simulink model "InversorDiesel"  (R2017a)
settings: Solver=VariableStepAuto  StartTime=0.0  StopTime=10.0  MaxStep=1e-4  RelTol=1e-3
values from neighbouring files (symbols this model uses):
  C1 = 1.1e-6    (= 1.1e-06)    [sistemacontrolado.m]
  L1 = 4.5e-3    (= 0.0045)    [sistemacontrolado.m]
  La = 3e-3    (= 0.003)    [sistemacontrolado.m]
  R1 = 1    [sistemacontrolado.m]
libraries: powerlib x17, instrumentlib x3, powerlib_extras x1, simulink x1
settings Model: Creator=MarioAndres  LastModifiedBy=Diego

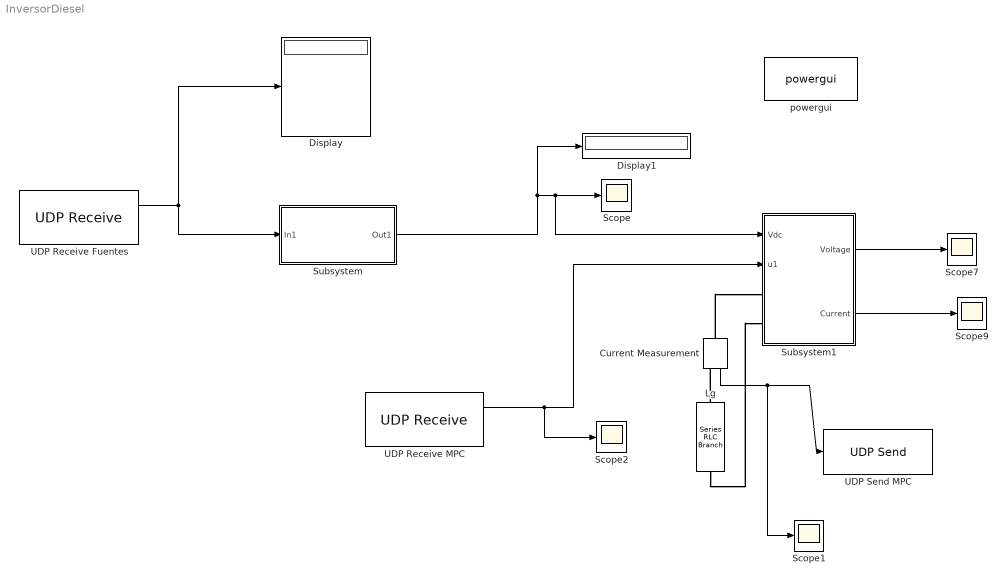
== system InversorDiesel ==
  Current Measurement : powerlib/Measurements/Current Measurement  PhasorSimulation=off  OutputType=Complex  PSBequivalent=0
  Display : Display
  Display1 : Display
  Lg : powerlib/Elements/Series RLC Branch  LConnTagsString=__new0  RConnTagsString=__new0  BranchType=L  Resistance=R1  Inductance=0.003  SetiL0=off  InitialCurrent=0  Capacitance=1e-6  Setx0=off  InitialVoltage=0  Measurements=None
  Scope{,1..2,7,9} (5 alike) : Scope
  Subsystem : Subsystem
  Subsystem1 : Subsystem
  UDP Receive Fuentes : instrumentlib/UDP Receive  Host=169.254.205.197  Port=51007  LocalPort=51006  DataSize="[6  1]"  EnableBlockingMode=off  Timeout=1  SampleTime=1  DataType=uint8  ByteOrder=BigEndian
      settings: SourceProductName=Instrument Control Toolbox
  UDP Receive MPC : instrumentlib/UDP Receive  Host=169.254.26.15  Port=51005  LocalPort=51004  DataSize="[6  1]"  EnableBlockingMode=off  Timeout=1  SampleTime=1  DataType=uint8  ByteOrder=BigEndian
      settings: SourceProductName=Instrument Control Toolbox
  UDP Send MPC : instrumentlib/UDP Send  Priority=2  Host=169.254.26.15  Port=51005  LocalPort=51004  EnableBlockingMode=on  ByteOrder=BigEndian
      settings: SourceProductName=Instrument Control Toolbox
  powergui : powerlib/powergui  SimulationMode=Continuous  SampleTime=1/60/10000  frequency=60  Iterations=50  frequencyindice=0  Pbase=100e6  ErrMax=1e-4  UnitsV=kV  UnitsW=MW  buscounter=0  FunctionMessages=off  echomessages=off  EnableUseOfTLC=off  CurrentSourceSwitches=off  DisableSnubberDevices=off  DisableRonSwitches=off  DisableVfSwitches=off  DisplayEquations=off  SolverType=Tustin/Backward Euler (TBE)  Interpol=off  ExternalGateDelay=off  methode=off  Ts=100  x0status=blocks  SPID=on  SwTol=0  HookPort=off  RestoreLinks=warning  ResistiveCurrentMeasurement=off  Frange=[0:2:500]  Ylog=off  Xlog=on  ShowGrid=off  save=off  variable=ZData  structure=sps1phPWM1_str  ZoomFFT=on  StartTime=0.1-2/60  cycles=2  DisplayStyle=1  fundamental=60  FreqAxis=off  MaxFrequency=5000  frequencyindicesteady=1  RmsSteady=1  display=off
  wires:
  UDP Receive Fuentes/1 -> Subsystem/1(In1), Display/1
  Subsystem1/1(Voltage) -> Scope7/1
  Subsystem1/2(Current) -> Scope9/1
  UDP Receive MPC/1 -> Scope2/1, Subsystem1/2(u1)
  Current Measurement/1 -> Scope1/1, UDP Send MPC/1
  Subsystem/1(Out1) -> Display1/1, Subsystem1/1(Vdc), Scope/1
  connections:
  Current Measurement/LConn1 -- Subsystem1/LConn1
  Lg/RConn1 -- Current Measurement/RConn1
  Lg/LConn1 -- Subsystem1/LConn2

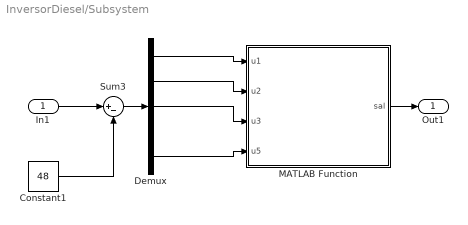
== system InversorDiesel/Subsystem ==
  In1 : Inport
  Constant1 : Constant  Value=48
  Demux : Demux  Outputs=5
  MATLAB Function : MATLAB Function  TreatAsAtomicUnit=on
  Sum3 : Sum  Inputs=|+-
  Out1 : Outport
  wires:
  Sum3/1 -> Demux/1
  In1/1 -> Sum3/1
  Constant1/1 -> Sum3/2
  Demux/1 -> MATLAB Function/1(u1)
  Demux/2 -> MATLAB Function/2(u2)
  Demux/3 -> MATLAB Function/3(u3)
  Demux/5 -> MATLAB Function/4(u5)
  MATLAB Function/1(sal) -> Out1/1

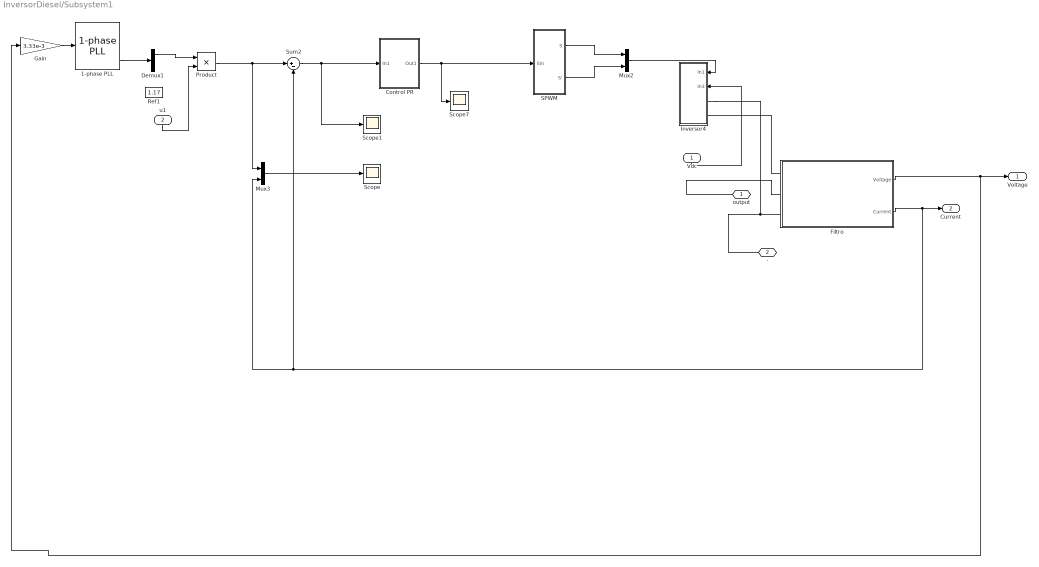
== system InversorDiesel/Subsystem1 ==
  Vdc : Inport
  u1 : Inport  Port=2
  1-phase PLL : powerlib_extras/Control  Blocks/1-phase PLL  Par_Init=[0 60]  ParK=[ 180 3200 1 ]  AGC=off
  Control PR : Subsystem
  Demux1 : Demux  Outputs=2
  Filtro : Subsystem
  Gain : Gain  Gain=3.33e-3
  Inversor4 : Subsystem
  Mux2 : Mux  Inputs=2
  Mux3 : Mux  Inputs=2
  Product : Product
  Ref1 : Constant  Value=1.17
  SPWM : Subsystem
  Scope : Scope
  Scope1 : Scope
  Scope7 : Scope
  Sum2 : Sum  Inputs=|+-
  output : PMIOPort  Port=1  Side=Left
  - : PMIOPort  Port=2  Side=Left
  Voltage : Outport
  Current : Outport  Port=2
  wires:
  Filtro/2(Current) -> Mux3/2, Sum2/2, Current/1
  Filtro/1(Voltage) -> Gain/1, Voltage/1
  1-phase PLL/3 -> Demux1/1
  Gain/1 -> 1-phase PLL/1
  Mux3/1 -> Scope/1
  Product/1 -> Mux3/1, Sum2/1
  Demux1/1 -> Product/1
  SPWM/1(S) -> Mux2/1
  SPWM/2(S') -> Mux2/2
  Mux2/1 -> Inversor4/1(In1)
  Vdc/1 -> Inversor4/2(In3)
  Control PR/1(Out1) -> Scope7/1, SPWM/1(Sin)
  Sum2/1 -> Scope1/1, Control PR/1(In1)
  u1/1 -> Product/2
  connections:
  output/RConn1 -- Filtro/LConn2
  -/RConn1 -- Inversor4/LConn1 -- Filtro/LConn3
  Filtro/LConn1 -- Inversor4/LConn2

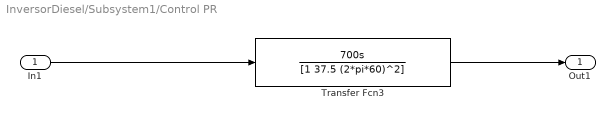
== system InversorDiesel/Subsystem1/Control PR ==
  In1 : Inport
  Transfer Fcn3 : TransferFcn  Numerator=[700 0]  Denominator=[1 37.5 (2*pi*60)^2]
  Out1 : Outport
  wires:
  In1/1 -> Transfer Fcn3/1
  Transfer Fcn3/1 -> Out1/1

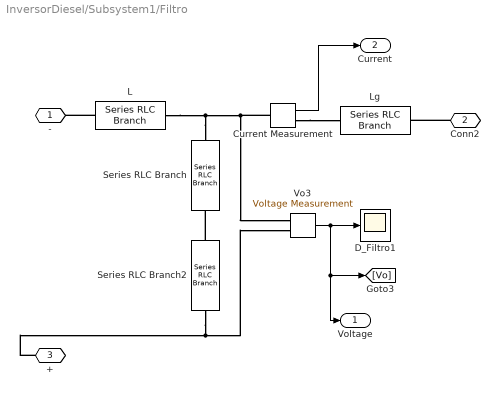
== system InversorDiesel/Subsystem1/Filtro ==
  Current Measurement : powerlib/Measurements/Current Measurement  PhasorSimulation=off  OutputType=Complex  PSBequivalent=0
  D_Filtro1 : Scope
  L : powerlib/Elements/Series RLC Branch  LConnTagsString=__new0  RConnTagsString=__new0  BranchType=RL  Resistance=0.01  Inductance=La  SetiL0=off  InitialCurrent=0  Capacitance=1e-6  Setx0=off  InitialVoltage=0  Measurements=None
  Lg : powerlib/Elements/Series RLC Branch  LConnTagsString=__new0  RConnTagsString=__new0  BranchType=RL  Resistance=R1  Inductance=L1  SetiL0=off  InitialCurrent=0  Capacitance=1e-6  Setx0=off  InitialVoltage=0  Measurements=None
  Series RLC Branch : powerlib/Elements/Series RLC Branch  LConnTagsString=__new0  RConnTagsString=__new0  BranchType=C  Resistance=10  Inductance=25e-3  SetiL0=off  InitialCurrent=0  Capacitance=C1  Setx0=on  InitialVoltage=0  Measurements=None
  Series RLC Branch2 : powerlib/Elements/Series RLC Branch  LConnTagsString=__new0  RConnTagsString=__new0  BranchType=R  Resistance=0.1  Inductance=25e-3  SetiL0=off  InitialCurrent=0  Capacitance=5.30e-3  Setx0=off  InitialVoltage=0  Measurements=None
  Vo3 : powerlib/Measurements/Voltage Measurement  PhasorSimulation=off  OutputType=Complex  PSBequivalent=0
  - : PMIOPort  Port=1  Side=Left
  Conn2 : PMIOPort  Port=2  Side=Left
  + : PMIOPort  Port=3  Side=Left
  Voltage : Outport
  Current : Outport  Port=2
  wires:
  Vo3/1 -> D_Filtro1/1, Voltage/1, [Vo]
  Current Measurement/1 -> Current/1
  connections:
  L/LConn1 -- -/RConn1
  Series RLC Branch/LConn1 -- Current Measurement/LConn1 -- Vo3/LConn1 -- L/RConn1
  Series RLC Branch2/LConn1 -- Series RLC Branch/RConn1
  Current Measurement/RConn1 -- Lg/LConn1
  Series RLC Branch2/RConn1 -- +/RConn1 -- Vo3/LConn2
  Conn2/RConn1 -- Lg/RConn1

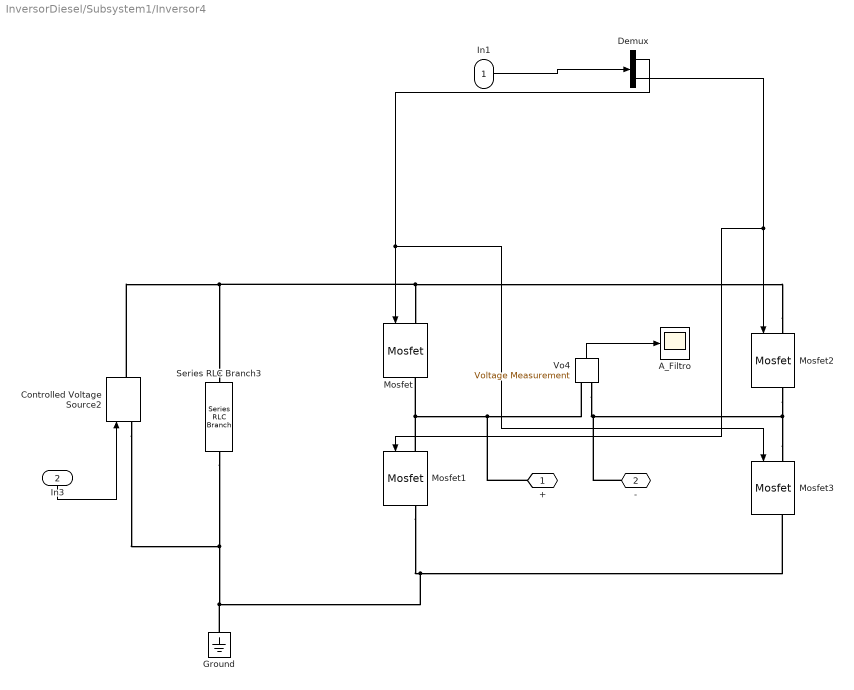
== system InversorDiesel/Subsystem1/Inversor4 ==
  In1 : Inport
  In3 : Inport  Port=2
  A_Filtro : Scope
  Controlled Voltage Source2 : powerlib/Electrical Sources/Controlled Voltage Source  Initialize=on  Source_Type=DC  Amplitude=0  Phase=0  Frequency=0  Measurements=None
  Demux : Demux  Outputs=2
  Ground : powerlib/Elements/Ground  LConnTagsString=a
  Mosfet{,1..3} (4 alike) : powerlib/Power Electronics/Mosfet  Ron=0.1  Lon=0  Rd=0.01  Vfd=0  IC=0  Rs=1e5  Cs=inf  Measurements=on
  Series RLC Branch3 : powerlib/Elements/Series RLC Branch  LConnTagsString=__new0  RConnTagsString=__new0  BranchType=RC  Resistance=1  Inductance=25e-3  SetiL0=off  InitialCurrent=0  Capacitance=2.2e-3  Setx0=off  InitialVoltage=0  Measurements=None
  Vo4 : powerlib/Measurements/Voltage Measurement  PhasorSimulation=off  OutputType=Complex  PSBequivalent=0
  + : PMIOPort  Port=1  Side=Left
  - : PMIOPort  Port=2  Side=Left
  wires:
  Vo4/1 -> A_Filtro/1
  Demux/1 -> Mosfet3/1, Mosfet/1
  Demux/2 -> Mosfet1/1, Mosfet2/1
  In3/1 -> Controlled Voltage Source2/1
  In1/1 -> Demux/1
  connections:
  Mosfet3/LConn1 -- -/RConn1 -- Vo4/LConn2 -- Mosfet2/RConn1
  Mosfet2/LConn1 -- Mosfet/LConn1 -- Controlled Voltage Source2/RConn1 -- Series RLC Branch3/LConn1
  Mosfet/RConn1 -- Mosfet1/LConn1 -- Vo4/LConn1 -- +/RConn1
  Mosfet1/RConn1 -- Series RLC Branch3/RConn1 -- Controlled Voltage Source2/LConn1 -- Ground/LConn1 -- Mosfet3/RConn1

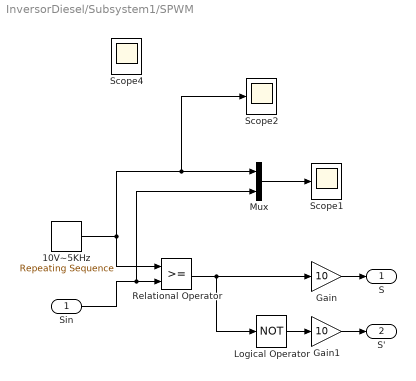
== system InversorDiesel/Subsystem1/SPWM ==
  Sin : Inport
  10V~5KHz : simulink/Sources/Repeating Sequence  rep_seq_t=[0 0.0001 0.0002]  rep_seq_y=[-10.5 10.5 -10.5]
  Gain : Gain  Gain=10
  Gain1 : Gain  Gain=10
  Logical Operator : Logic  Operator=NOT  AllPortsSameDT=off  OutDataTypeStr=boolean
  Mux : Mux  Inputs=2
  Relational Operator : RelationalOperator  OutDataTypeStr=boolean  RndMeth=Nearest
  Scope1 : Scope
  Scope2 : Scope
  Scope4 : Scope
  S : Outport
  S' : Outport  Port=2
  wires:
  10V~5KHz/1 -> Relational Operator/1, Mux/1, Scope2/1
  Relational Operator/1 -> Gain/1, Logical Operator/1
  Logical Operator/1 -> Gain1/1
  Gain/1 -> S/1
  Gain1/1 -> S'/1
  Mux/1 -> Scope1/1
  Sin/1 -> Relational Operator/2, Mux/2
  ? -> Scope4/1

== matlab function InversorDiesel/Subsystem/MATLAB Function ==
  data: u1 input; sal output; u2 input; u3 input; u5 input
function sal = fcn(u1,u2,u3,u5)
  if u1==0 && u2==0
      sal=u3+u5/10
  end
  if u1==0 && (u2~=0 || u2~=-3)
      sal=u2*10+u3+u5/10
  end
  if u1~=0 && u2~=0
      sal=u1*100+u2*10+u3+u5/10
  end
  
  if u2==-3
     sal=u3+u5/10
  end
  
  sal=u1*100+u2*10+u3+u5/10;
  
      
  

end
